simulink model "Main_Sim_Exp"  (R2020b)
settings: Solver=FixedStepAuto  StartTime=0.0  StopTime=6000  FixedStep=simParams.sample_time_s  RelTol=1e-3  EnableMultiTasking=on
values from neighbouring files (symbols this model uses):
  test_data = struct    [sim_init.m]
undefined symbols (not defined in the file or in its folder): simParams
libraries: dspstat3 x2, simulink_extras x2, aerolibutil x1
settings Model: Creator=devantormey  LastModifiedBy=Zach Daniel
settings DataIOCC: ReturnWorkspaceOutputs=off
settings OptimizationCC: DefaultParameterBehavior=Inlined  UseDivisionForNetSlopeComputation=on  UseFloatMulNetSlope=on  InlineInvariantSignals=on  PassReuseOutputArgsAs=Individual arguments  ZeroExternalMemoryAtStartup=off  ZeroInternalMemoryAtStartup=off  NoFixptDivByZeroProtection=on  EfficientFloat2IntCast=on  LifeSpan=1  OptimizeBlockOrder=speed  DifferentSizesBufferReuse=on  EfficientTunableParamExpr=on
settings DebuggingCC: ParameterTunabilityLossMsg=error  BusObjectLabelMismatch=error  SFUnexpectedBacktrackingDiag=warning  SFNoUnconditionalDefaultTransitionDiag=warning  ArithmeticOperatorsInVariantConditions=warning
settings HardwareCC: ProdBitPerPointer=32  ProdBitPerSizeT=32  ProdBitPerPtrDiffT=32  ProdLargestAtomicInteger=Long  ProdLargestAtomicFloat=Double  ProdWordSize=32  ProdLongLongMode=on  ProdHWDeviceType=NXP->Cortex-M4
settings SFSimCC: SimUseLocalCustomCode=off  MATLABDynamicMemAlloc=off  CustomCodeUndefinedFunction=UseInterfaceOnly
settings RTWCC: Description=Embedded Coder  SystemTargetFile=ert.tlc  TemplateMakefile=ert_default_tmf  GenerateReport=on  RTWUseLocalCustomCode=off  IncludeHyperlinkInReport=on  LaunchReport=on  GenerateTraceInfo=on  GenerateTraceReport=on  GenerateTraceReportSl=on  GenerateTraceReportSf=on  GenerateTraceReportEml=on  GenerateCodeMetricsReport=on
settings CodeAppCC: ForceParamTrailComments=on  IgnoreCustomStorageClasses=off  OperatorAnnotations=on  SimulinkDataObjDesc=on  SFDataObjDesc=on  CustomSymbolStrGlobalVar=rt$N$M  CustomSymbolStrType=$N$M  CustomSymbolStrFcn=$N$M$F  CustomSymbolStrMacro=$N$M  InsertBlockDesc=on
settings ERTTargetCC: GenerateSampleERTMain=on  IncludeMdlTerminateFcn=off  CombineSignalStateStructs=on  SupportComplex=off  SupportContinuousTime=on  SupportNonInlinedSFcns=on  InlinedParameterPlacement=NonHierarchical  ERTCustomFileTemplate=example_file_process.tlc
settings ConfigComp: CovMetricSettings=dw  CovSaveCumulativeToWorkspaceVar=on  CovSaveSingleToWorkspaceVar=on  CovExternalEMLEnable=off

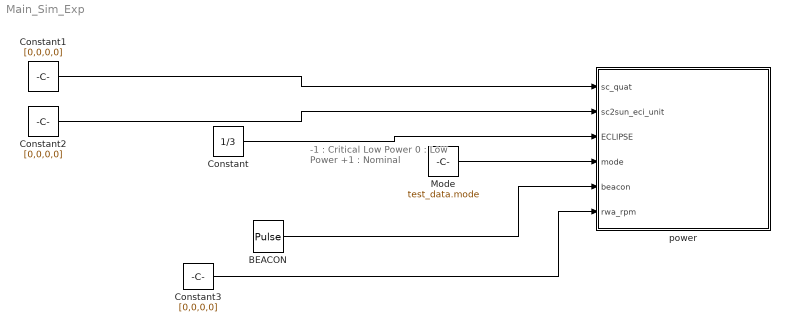
== system Main_Sim_Exp ==
  note: -1	: Critical Low Power
      |   0	: Low Power
      | +1	: Nominal
  BEACON : DiscretePulseGenerator  PulseType=Time based  Period=60  PulseWidth=100 * (1.0 / 60)
  Constant : Constant  Value=1/3
  Constant1 : Constant  Value=[0,0,0,0]
  Constant2 : Constant  Value=[0,0,0,0]
  Constant3 : Constant  Value=[0,0,0,0]
  Mode : Constant  Value=test_data.mode
  power : Subsystem
  wires:
  Mode/1 -> power/4(mode)
  BEACON/1 -> power/5(beacon)
  Constant/1 -> power/3(ECLIPSE)
  Constant1/1 -> power/1(sc_quat)
  Constant2/1 -> power/2(sc2sun_eci_unit)
  Constant3/1 -> power/6(rwa_rpm)

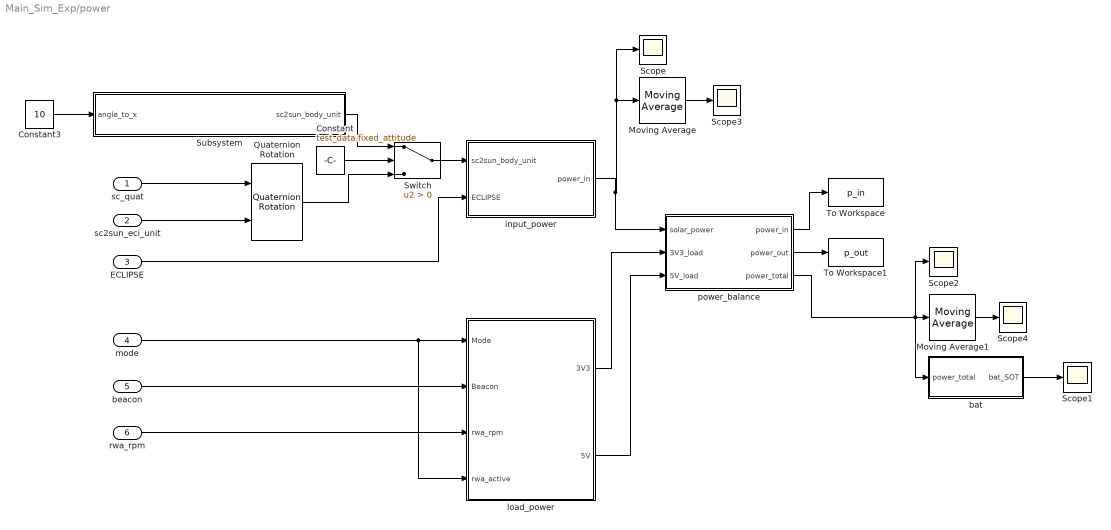
== system Main_Sim_Exp/power ==
  sc_quat : Inport
  sc2sun_eci_unit : Inport  Port=2
  ECLIPSE : Inport  Port=3
  mode : Inport  Port=4
  beacon : Inport  Port=5
  rwa_rpm : Inport  Port=6
  Constant : Constant  Value=test_data.fixed_attitude
  Constant3 : Constant  Value=10
  Moving Average : dspstat3/Moving Average  Method=Exponential weighting  ForgettingFactorPort=off  SpecifyWindowLength=on  WindowLength=4  ForgettingFactor=1.0  SimulateUsing=Code generation
  Moving Average1 : dspstat3/Moving Average  Method=Exponential weighting  ForgettingFactorPort=off  SpecifyWindowLength=on  WindowLength=4  ForgettingFactor=1.0  SimulateUsing=Code generation
  Quaternion Rotation : aerolibutil/Quaternion Rotation
  Scope{,1..4} (5 alike) : Scope
  Subsystem : Subsystem
  Switch : Switch  Criteria=u2 > Threshold
  To Workspace : ToWorkspace  VariableName=p_in  SampleTime=-1
  To Workspace1 : ToWorkspace  VariableName=p_out  SampleTime=-1
  bat : Subsystem
  input_power : Subsystem
  load_power : Subsystem
  power_balance : Subsystem
  wires:
  load_power/1(3V3) -> power_balance/2("3V3_load ")
  input_power/1(power_in) -> power_balance/1(solar_power), Moving Average/1, Scope/1
  rwa_rpm/1 -> load_power/3(rwa_rpm)
  mode/1 -> load_power/4(rwa_active), load_power/1(Mode)
  beacon/1 -> load_power/2(Beacon)
  Moving Average1/1 -> Scope4/1
  load_power/2(5V) -> power_balance/3(5V_load)
  bat/1(bat_SOT) -> Scope1/1
  Moving Average/1 -> Scope3/1
  sc_quat/1 -> Quaternion Rotation/1
  sc2sun_eci_unit/1 -> Quaternion Rotation/2
  ECLIPSE/1 -> input_power/2(ECLIPSE)
  power_balance/3(power_total) -> Scope2/1, bat/1(power_total), Moving Average1/1
  power_balance/1(power_in) -> To Workspace/1
  power_balance/2(power_out) -> To Workspace1/1
  Constant3/1 -> Subsystem/1(angle_to_x)
  Constant/1 -> Switch/2
  Subsystem/1(sc2sun_body_unit) -> Switch/1
  Quaternion Rotation/1 -> Switch/3
  Switch/1 -> input_power/1(sc2sun_body_unit)

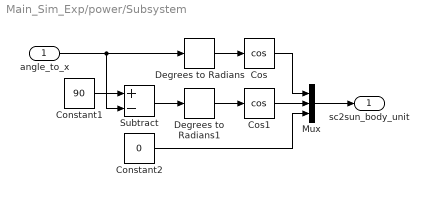
== system Main_Sim_Exp/power/Subsystem ==
  angle_to_x : Inport
  Constant1 : Constant  Value=90
  Constant2 : Constant  Value=0
  Cos : Trigonometry  Operator=cos
  Cos1 : Trigonometry  Operator=cos
  Degrees to Radians : simulink_extras/Transformations/Degrees to Radians
  Degrees to Radians1 : simulink_extras/Transformations/Degrees to Radians
  Mux : Mux  Inputs=3
  Subtract : Sum  Inputs=+-
  sc2sun_body_unit : Outport  VectorParamsAs1DForOutWhenUnconnected=off
  wires:
  Subtract/1 -> Degrees to Radians1/1
  Constant2/1 -> Mux/3
  Cos1/1 -> Mux/2
  Degrees to Radians1/1 -> Cos1/1
  Degrees to Radians/1 -> Cos/1
  Cos/1 -> Mux/1
  Mux/1 -> sc2sun_body_unit/1
  Constant1/1 -> Subtract/1
  angle_to_x/1 -> Subtract/2, Degrees to Radians/1

== system Main_Sim_Exp/power/bat ==
  power_total : Inport
  Constant4 : Constant  Value=1/(60*60)
  Constant5 : Constant  Value=20000
  Divide : Product  Inputs=*/
  Integrator : Integrator  InitialCondition=20000  LimitOutput=on  UpperSaturationLimit=20000  LowerSaturationLimit=0
  Product : Product
  bat_SOT : Outport  VectorParamsAs1DForOutWhenUnconnected=off
  wires:
  Constant4/1 -> Product/2
  Constant5/1 -> Divide/2
  power_total/1 -> Product/1
  Product/1 -> Integrator/1
  Integrator/1 -> Divide/1
  Divide/1 -> bat_SOT/1

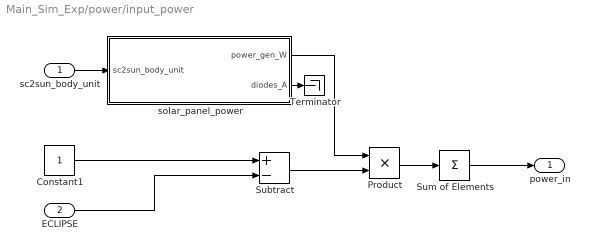
== system Main_Sim_Exp/power/input_power ==
  sc2sun_body_unit : Inport
  ECLIPSE : Inport  Port=2
  Constant1 : Constant
  Product : Product
  Subtract : Sum  Inputs=+-
  Sum of Elements : Sum  Inputs=+
  Terminator : Terminator
  solar_panel_power : MATLAB Function  TreatAsAtomicUnit=on
  power_in : Outport  VectorParamsAs1DForOutWhenUnconnected=off
  wires:
  Product/1 -> Sum of Elements/1
  solar_panel_power/2(diodes_A) -> Terminator/1
  solar_panel_power/1(power_gen_W) -> Product/1
  Sum of Elements/1 -> power_in/1
  sc2sun_body_unit/1 -> solar_panel_power/1(sc2sun_body_unit)
  Constant1/1 -> Subtract/1
  ECLIPSE/1 -> Subtract/2
  Subtract/1 -> Product/2

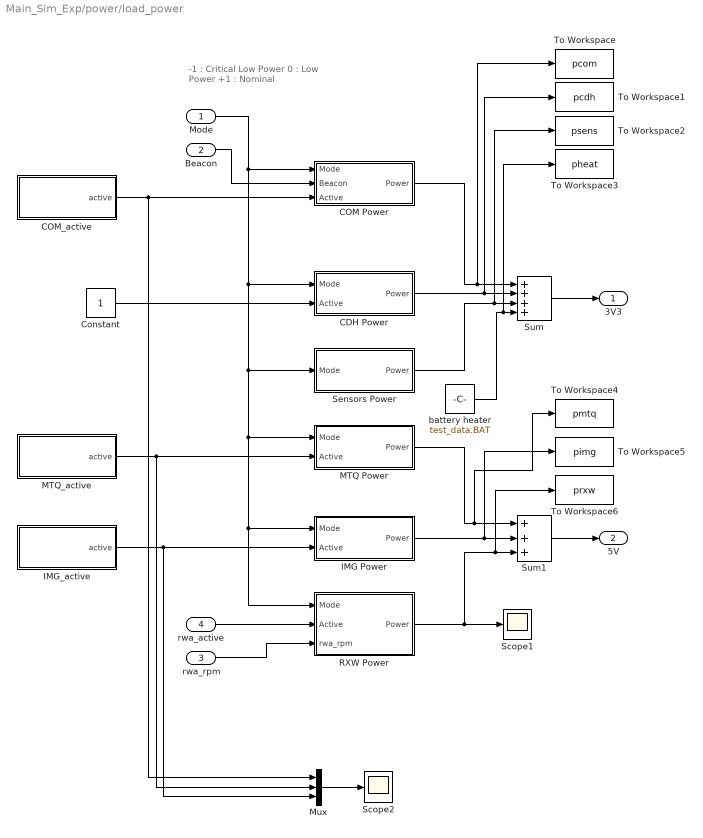
== system Main_Sim_Exp/power/load_power ==
  note: -1	: Critical Low Power
      |   0	: Low Power
      | +1	: Nominal
  Mode : Inport
  Beacon : Inport  Port=2
  rwa_rpm : Inport  Port=3
  rwa_active : Inport  Port=4
  CDH Power : Subsystem
  COM Power : Subsystem
  COM_active : Subsystem
  Constant : Constant
  IMG Power : Subsystem
  IMG_active : Subsystem
  MTQ Power : Subsystem
  MTQ_active : Subsystem
  Mux : Mux  Inputs=3
  RXW Power : Subsystem
  Scope1 : Scope
  Scope2 : Scope
  Sensors Power : Subsystem
  Sum : Sum  Inputs=++++
  Sum1 : Sum  Inputs=+++
  To Workspace : ToWorkspace  VariableName=pcom  SampleTime=-1
  To Workspace1 : ToWorkspace  VariableName=pcdh  SampleTime=-1
  To Workspace2 : ToWorkspace  VariableName=psens  SampleTime=-1
  To Workspace3 : ToWorkspace  VariableName=pheat  SampleTime=-1
  To Workspace4 : ToWorkspace  VariableName=pmtq  SampleTime=-1
  To Workspace5 : ToWorkspace  VariableName=pimg  SampleTime=-1
  To Workspace6 : ToWorkspace  VariableName=prxw  SampleTime=-1
  battery heater : Constant  Value=test_data.BAT
  3V3 : Outport  VectorParamsAs1DForOutWhenUnconnected=off
  5V : Outport  Port=2  VectorParamsAs1DForOutWhenUnconnected=off
  wires:
  Mode/1 -> RXW Power/1(Mode), IMG Power/1(Mode), MTQ Power/1(Mode), Sensors Power/1(Mode), CDH Power/1(Mode), COM Power/1(Mode)
  Beacon/1 -> COM Power/2(Beacon)
  rwa_active/1 -> RXW Power/2(Active)
  CDH Power/1(Power) -> Sum/2, To Workspace1/1
  COM Power/1(Power) -> Sum/1, To Workspace/1
  Sensors Power/1(Power) -> Sum/3, To Workspace2/1
  IMG Power/1(Power) -> To Workspace5/1, Sum1/2
  RXW Power/1(Power) -> Scope1/1, To Workspace6/1, Sum1/3
  Sum/1 -> 3V3/1
  Sum1/1 -> 5V/1
  battery heater/1 -> To Workspace3/1, Sum/4
  rwa_rpm/1 -> RXW Power/3(rwa_rpm)
  MTQ Power/1(Power) -> To Workspace4/1, Sum1/1
  IMG_active/1(active) -> Mux/3, IMG Power/2(Active)
  MTQ_active/1(active) -> Mux/2, MTQ Power/2(Active)
  Constant/1 -> CDH Power/2(Active)
  COM_active/1(active) -> Mux/1, COM Power/3("Active ")
  Mux/1 -> Scope2/1

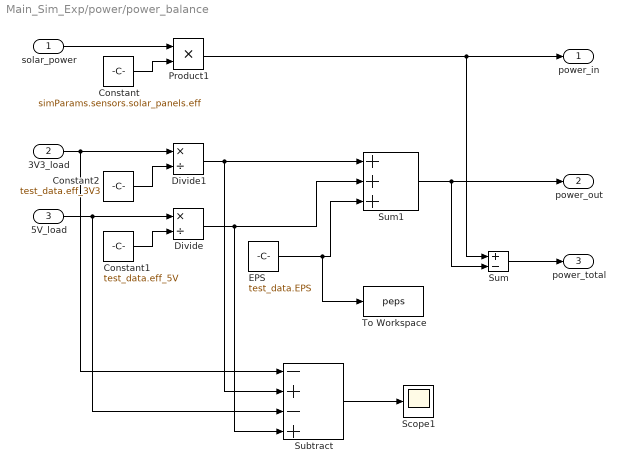
== system Main_Sim_Exp/power/power_balance ==
  solar_power : Inport
  "3V3_load " : Inport  Port=2
  5V_load : Inport  Port=3
  Constant : Constant  Value=simParams.sensors.solar_panels.eff
  Constant1 : Constant  Value=test_data.eff_5V
  Constant2 : Constant  Value=test_data.eff_3V3
  Divide : Product  Inputs=*/
  Divide1 : Product  Inputs=*/
  EPS : Constant  Value=test_data.EPS
  Product1 : Product
  Scope1 : Scope
  Subtract : Sum  Inputs=-+-+
  Sum : Sum  Inputs=+-
  Sum1 : Sum  Inputs=+++
  To Workspace : ToWorkspace  VariableName=peps  SampleTime=-1
  power_in : Outport  VectorParamsAs1DForOutWhenUnconnected=off
  power_out : Outport  Port=2  VectorParamsAs1DForOutWhenUnconnected=off
  power_total : Outport  Port=3  VectorParamsAs1DForOutWhenUnconnected=off
  wires:
  solar_power/1 -> Product1/1
  Constant/1 -> Product1/2
  5V_load/1 -> Subtract/3, Divide/1
  Constant1/1 -> Divide/2
  Constant2/1 -> Divide1/2
  "3V3_load "/1 -> Subtract/1, Divide1/1
  Divide1/1 -> Sum1/1, Subtract/2
  Product1/1 -> Sum/1, power_in/1
  Divide/1 -> Sum1/2, Subtract/4
  Sum1/1 -> Sum/2, power_out/1
  EPS/1 -> To Workspace/1, Sum1/3
  Subtract/1 -> Scope1/1
  Sum/1 -> power_total/1

== system Main_Sim_Exp/power/load_power/CDH Power ==
  Mode : Inport
  Active : Inport  Port=2
  Constant : Constant  Value=-1
  Constant1 : Constant  Value=test_data.CDH_Idle
  Constant2 : Constant  Value=test_data.CDH_Active
  GreaterThan : RelationalOperator  OutDataTypeStr=boolean  RndMeth=Simplest
  Logical Operator : Logic  AllPortsSameDT=off  OutDataTypeStr=boolean
  Switch : Switch  Criteria=u2 > Threshold
  Power : Outport
  wires:
  Constant/1 -> GreaterThan/2
  Mode/1 -> GreaterThan/1
  GreaterThan/1 -> Logical Operator/1
  Active/1 -> Logical Operator/2
  Logical Operator/1 -> Switch/2
  Switch/1 -> Power/1
  Constant2/1 -> Switch/1
  Constant1/1 -> Switch/3

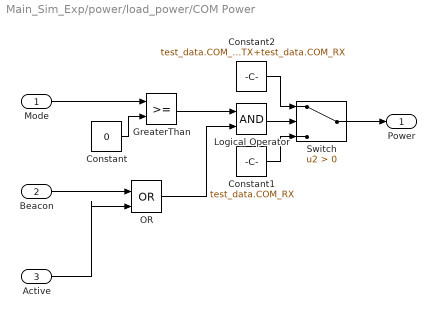
== system Main_Sim_Exp/power/load_power/COM Power ==
  Mode : Inport
  Beacon : Inport  Port=2
  "Active " : Inport  Port=3
  Constant : Constant  Value=0
  Constant1 : Constant  Value=test_data.COM_RX
  Constant2 : Constant  Value=test_data.COM_TX+test_data.COM_RX
  GreaterThan : RelationalOperator  OutDataTypeStr=boolean  RndMeth=Simplest
  Logical Operator : Logic  AllPortsSameDT=off  OutDataTypeStr=boolean
  OR : Logic  Operator=OR  IconShape=distinctive  AllPortsSameDT=off  OutDataTypeStr=boolean
  Switch : Switch  Criteria=u2 > Threshold
  Power : Outport
  wires:
  Constant/1 -> GreaterThan/2
  Mode/1 -> GreaterThan/1
  GreaterThan/1 -> Logical Operator/1
  Constant2/1 -> Switch/1
  Constant1/1 -> Switch/3
  Logical Operator/1 -> Switch/2
  Switch/1 -> Power/1
  Beacon/1 -> OR/1
  "Active "/1 -> OR/2
  OR/1 -> Logical Operator/2

== system Main_Sim_Exp/power/load_power/COM_active ==
  Constant : Constant  Value=0
  Constant1 : Constant  Value=test_data.com_en
  Product4 : Product
  Step6 : Step  Time=test_data.com_start  SampleTime=0
  Step7 : Step  Time=test_data.com_end  Before=1  After=0  SampleTime=0
  Switch : Switch  Criteria=u2 > Threshold
  active : Outport  VectorParamsAs1DForOutWhenUnconnected=off
  wires:
  Product4/1 -> Switch/1
  Step7/1 -> Product4/2
  Step6/1 -> Product4/1
  Constant/1 -> Switch/3
  Constant1/1 -> Switch/2
  Switch/1 -> active/1

== system Main_Sim_Exp/power/load_power/IMG Power ==
  Mode : Inport
  Active : Inport  Port=2
  Constant : Constant
  Constant1 : Constant  Value=test_data.IMG_Idle
  Constant2 : Constant  Value=test_data.IMG_Active
  GreaterThan : RelationalOperator  OutDataTypeStr=boolean  RndMeth=Simplest
  Logical Operator : Logic  AllPortsSameDT=off  OutDataTypeStr=boolean
  Switch : Switch  Criteria=u2 > Threshold
  Power : Outport
  wires:
  Constant/1 -> GreaterThan/2
  Mode/1 -> GreaterThan/1
  GreaterThan/1 -> Logical Operator/1
  Active/1 -> Logical Operator/2
  Logical Operator/1 -> Switch/2
  Constant2/1 -> Switch/1
  Constant1/1 -> Switch/3
  Switch/1 -> Power/1

== system Main_Sim_Exp/power/load_power/IMG_active ==
  Constant : Constant  Value=0
  Constant1 : Constant  Value=test_data.img_en
  Product4 : Product
  Step6 : Step  Time=test_data.img_start  SampleTime=0
  Step7 : Step  Time=test_data.img_end  Before=1  After=0  SampleTime=0
  Switch : Switch  Criteria=u2 > Threshold
  active : Outport  VectorParamsAs1DForOutWhenUnconnected=off
  wires:
  Product4/1 -> Switch/1
  Step7/1 -> Product4/2
  Step6/1 -> Product4/1
  Constant/1 -> Switch/3
  Constant1/1 -> Switch/2
  Switch/1 -> active/1

== system Main_Sim_Exp/power/load_power/MTQ Power ==
  Mode : Inport
  Active : Inport  Port=2
  Constant : Constant
  Constant1 : Constant  Value=test_data.MTQ_Active
  Constant2 : Constant  Value=test_data.MTQ_Idle
  GreaterThan : RelationalOperator  OutDataTypeStr=boolean  RndMeth=Simplest
  Logical Operator : Logic  AllPortsSameDT=off  OutDataTypeStr=boolean
  Switch : Switch  Criteria=u2 > Threshold
  Power : Outport
  wires:
  Constant/1 -> GreaterThan/2
  Mode/1 -> GreaterThan/1
  GreaterThan/1 -> Logical Operator/1
  Constant1/1 -> Switch/1
  Active/1 -> Logical Operator/2
  Logical Operator/1 -> Switch/2
  Constant2/1 -> Switch/3
  Switch/1 -> Power/1

== system Main_Sim_Exp/power/load_power/MTQ_active ==
  Constant : Constant  Value=0
  Constant1 : Constant  Value=test_data.mtq_en
  Product4 : Product
  Step6 : Step  Time=test_data.mtq_start  SampleTime=0
  Step7 : Step  Time=test_data.mtq_end  Before=1  After=0  SampleTime=0
  Switch : Switch  Criteria=u2 > Threshold
  active : Outport  VectorParamsAs1DForOutWhenUnconnected=off
  wires:
  Product4/1 -> Switch/1
  Step7/1 -> Product4/2
  Step6/1 -> Product4/1
  Constant/1 -> Switch/3
  Constant1/1 -> Switch/2
  Switch/1 -> active/1

== system Main_Sim_Exp/power/load_power/RXW Power ==
  Mode : Inport
  Active : Inport  Port=2
  rwa_rpm : Inport  Port=3
  Subsystem1 : Subsystem
  Power : Outport
  wires:
  Mode/1 -> Subsystem1/1(Mode)
  Active/1 -> Subsystem1/2(Active)
  rwa_rpm/1 -> Subsystem1/3(RPM)
  Subsystem1/1(Power) -> Power/1

== system Main_Sim_Exp/power/load_power/Sensors Power ==
  Mode : Inport
  Constant : Constant  Value=0
  Constant1 : Constant  Value=test_data.SEN_AVG
  GreaterThan : RelationalOperator  OutDataTypeStr=boolean  RndMeth=Simplest
  Product1 : Product
  Power : Outport
  wires:
  Constant/1 -> GreaterThan/2
  Mode/1 -> GreaterThan/1
  GreaterThan/1 -> Product1/2
  Constant1/1 -> Product1/1
  Product1/1 -> Power/1

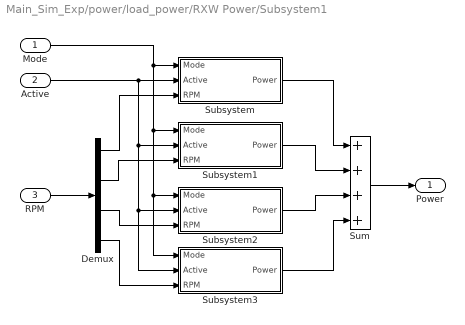
== system Main_Sim_Exp/power/load_power/RXW Power/Subsystem1 ==
  Mode : Inport
  Active : Inport  Port=2
  RPM : Inport  Port=3
  Demux : Demux
  Subsystem : Subsystem
  Subsystem1 : Subsystem
  Subsystem2 : Subsystem
  Subsystem3 : Subsystem
  Sum : Sum  Inputs=++++
  Power : Outport  VectorParamsAs1DForOutWhenUnconnected=off
  wires:
  RPM/1 -> Demux/1
  Mode/1 -> Subsystem3/1(Mode), Subsystem2/1(Mode), Subsystem1/1(Mode), Subsystem/1(Mode)
  Active/1 -> Subsystem3/2(Active), Subsystem2/2(Active), Subsystem1/2(Active), Subsystem/2(Active)
  Demux/1 -> Subsystem/3(RPM)
  Demux/2 -> Subsystem1/3(RPM)
  Demux/3 -> Subsystem2/3(RPM)
  Demux/4 -> Subsystem3/3(RPM)
  Subsystem1/1(Power) -> Sum/2
  Subsystem2/1(Power) -> Sum/3
  Subsystem3/1(Power) -> Sum/4
  Subsystem/1(Power) -> Sum/1
  Sum/1 -> Power/1

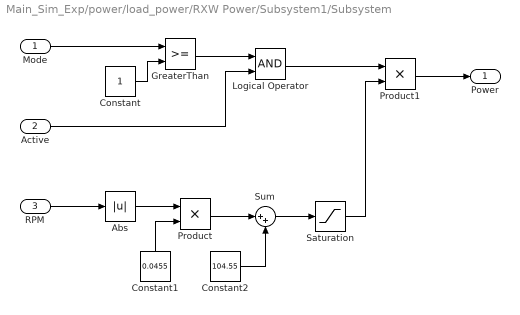
== system Main_Sim_Exp/power/load_power/RXW Power/Subsystem1/Subsystem ==
  Mode : Inport
  Active : Inport  Port=2
  RPM : Inport  Port=3
  Abs : Abs
  Constant : Constant
  Constant1 : Constant  Value=0.0455
  Constant2 : Constant  Value=104.55
  GreaterThan : RelationalOperator  OutDataTypeStr=boolean  RndMeth=Simplest
  Logical Operator : Logic  AllPortsSameDT=off  OutDataTypeStr=boolean
  Product : Product
  Product1 : Product
  Saturation : Saturate  UpperLimit=inf  LowerLimit=150
  Sum : Sum  Inputs=|++
  Power : Outport  VectorParamsAs1DForOutWhenUnconnected=off
  wires:
  Constant1/1 -> Product/2
  Logical Operator/1 -> Product1/1
  GreaterThan/1 -> Logical Operator/1
  Mode/1 -> GreaterThan/1
  Active/1 -> Logical Operator/2
  Constant/1 -> GreaterThan/2
  Product/1 -> Sum/1
  Constant2/1 -> Sum/2
  Sum/1 -> Saturation/1
  RPM/1 -> Abs/1
  Abs/1 -> Product/1
  Saturation/1 -> Product1/2
  Product1/1 -> Power/1

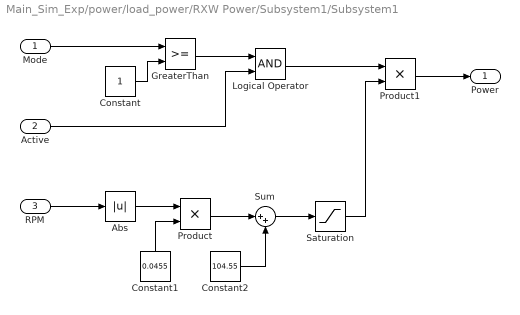
== system Main_Sim_Exp/power/load_power/RXW Power/Subsystem1/Subsystem1 ==
  Mode : Inport
  Active : Inport  Port=2
  RPM : Inport  Port=3
  Abs : Abs
  Constant : Constant
  Constant1 : Constant  Value=0.0455
  Constant2 : Constant  Value=104.55
  GreaterThan : RelationalOperator  OutDataTypeStr=boolean  RndMeth=Simplest
  Logical Operator : Logic  AllPortsSameDT=off  OutDataTypeStr=boolean
  Product : Product
  Product1 : Product
  Saturation : Saturate  UpperLimit=inf  LowerLimit=150
  Sum : Sum  Inputs=|++
  Power : Outport  VectorParamsAs1DForOutWhenUnconnected=off
  wires:
  Constant1/1 -> Product/2
  Logical Operator/1 -> Product1/1
  GreaterThan/1 -> Logical Operator/1
  Mode/1 -> GreaterThan/1
  Active/1 -> Logical Operator/2
  Constant/1 -> GreaterThan/2
  Product/1 -> Sum/1
  Constant2/1 -> Sum/2
  Sum/1 -> Saturation/1
  RPM/1 -> Abs/1
  Abs/1 -> Product/1
  Saturation/1 -> Product1/2
  Product1/1 -> Power/1

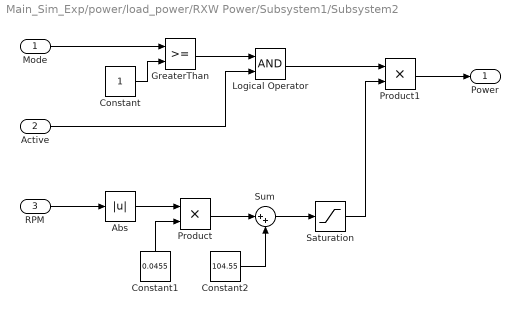
== system Main_Sim_Exp/power/load_power/RXW Power/Subsystem1/Subsystem2 ==
  Mode : Inport
  Active : Inport  Port=2
  RPM : Inport  Port=3
  Abs : Abs
  Constant : Constant
  Constant1 : Constant  Value=0.0455
  Constant2 : Constant  Value=104.55
  GreaterThan : RelationalOperator  OutDataTypeStr=boolean  RndMeth=Simplest
  Logical Operator : Logic  AllPortsSameDT=off  OutDataTypeStr=boolean
  Product : Product
  Product1 : Product
  Saturation : Saturate  UpperLimit=inf  LowerLimit=150
  Sum : Sum  Inputs=|++
  Power : Outport  VectorParamsAs1DForOutWhenUnconnected=off
  wires:
  Constant1/1 -> Product/2
  Logical Operator/1 -> Product1/1
  GreaterThan/1 -> Logical Operator/1
  Mode/1 -> GreaterThan/1
  Active/1 -> Logical Operator/2
  Constant/1 -> GreaterThan/2
  Product/1 -> Sum/1
  Constant2/1 -> Sum/2
  Sum/1 -> Saturation/1
  RPM/1 -> Abs/1
  Abs/1 -> Product/1
  Saturation/1 -> Product1/2
  Product1/1 -> Power/1

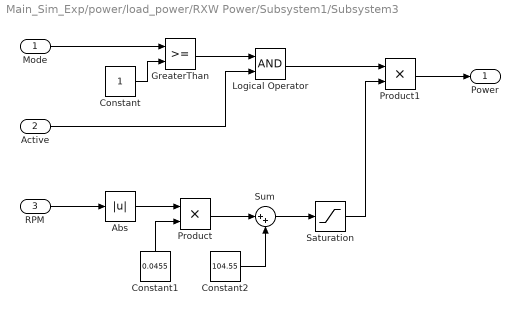
== system Main_Sim_Exp/power/load_power/RXW Power/Subsystem1/Subsystem3 ==
  Mode : Inport
  Active : Inport  Port=2
  RPM : Inport  Port=3
  Abs : Abs
  Constant : Constant
  Constant1 : Constant  Value=0.0455
  Constant2 : Constant  Value=104.55
  GreaterThan : RelationalOperator  OutDataTypeStr=boolean  RndMeth=Simplest
  Logical Operator : Logic  AllPortsSameDT=off  OutDataTypeStr=boolean
  Product : Product
  Product1 : Product
  Saturation : Saturate  UpperLimit=inf  LowerLimit=150
  Sum : Sum  Inputs=|++
  Power : Outport  VectorParamsAs1DForOutWhenUnconnected=off
  wires:
  Constant1/1 -> Product/2
  Logical Operator/1 -> Product1/1
  GreaterThan/1 -> Logical Operator/1
  Mode/1 -> GreaterThan/1
  Active/1 -> Logical Operator/2
  Constant/1 -> GreaterThan/2
  Product/1 -> Sum/1
  Constant2/1 -> Sum/2
  Sum/1 -> Saturation/1
  RPM/1 -> Abs/1
  Abs/1 -> Product/1
  Saturation/1 -> Product1/2
  Product1/1 -> Power/1

== matlab function Main_Sim_Exp/power/input_power/solar_panel_power ==
  data: sc2sun_body_unit input; power_gen_W output; simParams parameter; diodes_A output
function [power_gen_W,diodes_A] = get_power_gen(sc2sun_body_unit,simParams)
%GET_POWER_GEN
% 
% get_power_gen(sc2sun_body_unit,simParams) computes the total power being
% generated by the solar panels located on each of face. Assumes power
% generation is proportional to the square of the cosine of the incidence 
% angle to the sun, and can generate a maximum of 'maxPower' for each face.
%
% Assumes there are solar panels on all 6 sides of cuboid s/c, but fewer
% faces can be modeled by setting the 'maxPower' of those faces to zero.
% ORDER OF FACES: [ +x, -x, +y, -y, +z, -z ]
%
% This function also outputs the current reading from the photodiode on
% each face in Amps as diodes_A
%
% T. Reynolds
%#codegen

power_gen_W = zeros(6,1);
diodes_A    = zeros(6,1);
normals     = simParams.sensors.solar_panels.normals;
maxPower    = simParams.sensors.solar_panels.maxPower;
I_out_ApW   = simParams.sensors.photodiodes.I_out_ApW;

for k = 1:6
   % compute cos(incidence)
   sdotf = dot(normals(:,k),sc2sun_body_unit);
   cinc  = saturate(sdotf);
   incidence = acos(cinc);
   
   if incidence > 0.698132 % greater than 40 degrees
       factor = (-0.369 * cinc^3) + (0.637 * cinc^2) + (0.75 * cinc) -0.015;
   else
       factor = cinc;
   end
       
   if factor < 0
       factor = 0;
   end
   % compute power generated on ith face
   power_gen_W(k) = maxPower(k) * factor; %* cinc * cinc;
   
   % compute photodiode current
   diodes_A(k) = power_gen_W(k) * I_out_ApW; 
end

end

function y = saturate(x)
    if( x < 0 )
        y = 0.0;
    elseif( x >= 1.0 )
        y = 1.0;
    else
        y = x;
    end
end
